simulink model "connected_tanks_simulink"  (R2020a)
settings: Solver=VariableStepAuto  StartTime=0.0  StopTime=300  RelTol=1e-3
values from neighbouring files (symbols this model uses):
  a1 = 1.78    [connected_tanks.m]
  A1 = 15.518    [connected_tanks.m]
  a2 = 1.78    [connected_tanks.m]
  A2 = 15.518    [connected_tanks.m]
  g = 981    [connected_tanks.m]
  K0 = 5    [connected_tanks.m]
  K1 = 5    [connected_tanks.m]
  Kd = 1    [connected_tanks.m]
  Ke = 1    [connected_tanks.m]
  Km = 4.6    [connected_tanks.m]
libraries: fuzblock x2, simulink x1
settings Model: Creator=paulo  LastModifiedBy=paulo

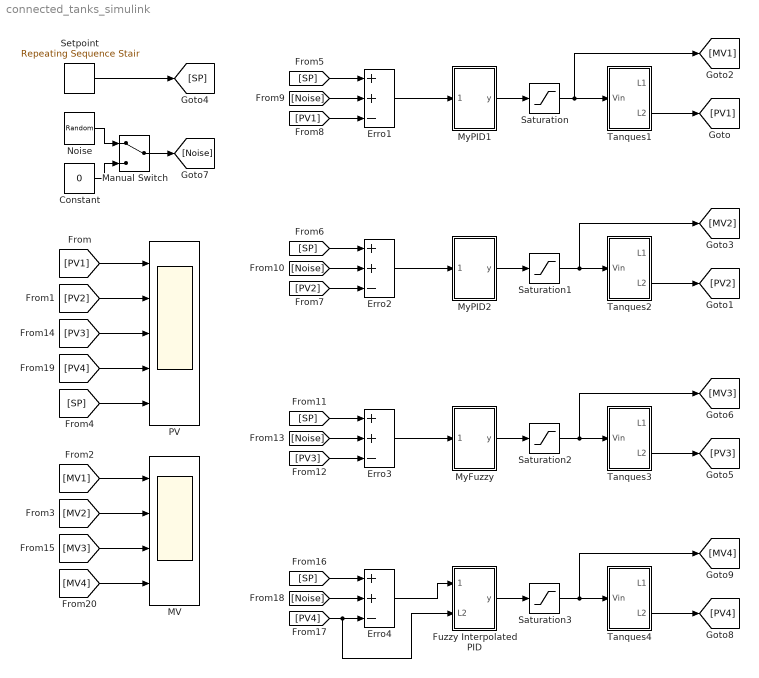
== system connected_tanks_simulink ==
  Constant : Constant  Value=0
  Erro{1..4} (4 alike) : Sum  Inputs=++-
  Fuzzy Interpolated PID : Subsystem
  MV : Scope  NumInputPorts=4
  Manual Switch : ManualSwitch
  MyFuzzy : Subsystem
  MyPID1 : Subsystem
  MyPID2 : Subsystem
  Noise : UniformRandomNumber  Minimum=-.5  Maximum=+.5  SampleTime=.5
  PV : Scope  NumInputPorts=5
  Saturation{,1..3} (4 alike) : Saturate  UpperLimit=120  LowerLimit=0
  Setpoint : simulink/Sources/Repeating Sequence Stair  OutValues=[5 20 15].'  tsamp=100  OutMin=[]  OutMax=[]  OutDataTypeStr=double  OutputDataTypeScalingMode=double  OutDataType=fixdt(0,8)  ConRadixGroup=Best Precision: Vector-wise  OutScaling=2^-12
  Tanques1 : Subsystem
  Tanques2 : Subsystem
  Tanques3 : Subsystem
  Tanques4 : Subsystem
  wires:
  Tanques1/2(L2) -> [PV1]
  Erro1/1 -> MyPID1/1(erro)
  MyPID1/1(y) -> Saturation/1
  Erro2/1 -> MyPID2/1(erro)
  Tanques2/2(L2) -> [PV2]
  [MV1] -> MV/1
  [MV2] -> MV/2
  Saturation/1 -> [MV1], Tanques1/1(Vin)
  Noise/1 -> Manual Switch/1
  Constant/1 -> Manual Switch/2
  MyPID2/1(y) -> Saturation1/1
  Saturation1/1 -> [MV2], Tanques2/1(Vin)
  Setpoint/1 -> [SP]
  [SP] -> Erro1/1
  [SP] -> Erro2/1
  Erro3/1 -> MyFuzzy/1(erro)
  MyFuzzy/1(y) -> Saturation2/1
  Tanques3/2(L2) -> [PV3]
  Saturation2/1 -> [MV3], Tanques3/1(Vin)
  [SP] -> Erro3/1
  [PV1] -> Erro1/3
  [Noise] -> Erro1/2
  Manual Switch/1 -> [Noise]
  [PV3] -> Erro3/3
  [Noise] -> Erro3/2
  [PV2] -> Erro2/3
  [Noise] -> Erro2/2
  [MV3] -> MV/3
  Tanques4/2(L2) -> [PV4]
  Saturation3/1 -> [MV4], Tanques4/1(Vin)
  [SP] -> Erro4/1
  Fuzzy Interpolated PID/1(y) -> Saturation3/1
  [PV4] -> Fuzzy Interpolated PID/2(L2), Erro4/3
  [Noise] -> Erro4/2
  Erro4/1 -> Fuzzy Interpolated PID/1(erro)
  [MV4] -> MV/4
  [PV1] -> PV/1
  [PV2] -> PV/2
  [PV3] -> PV/3
  [PV4] -> PV/4
  [SP] -> PV/5

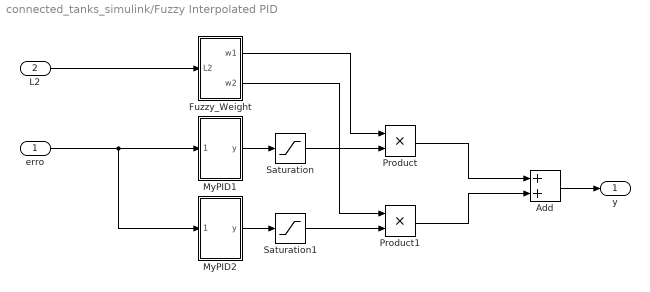
== system connected_tanks_simulink/Fuzzy Interpolated PID ==
  erro : Inport
  L2 : Inport  Port=2
  Add : Sum
  Fuzzy_Weight : Subsystem
  MyPID1 : Subsystem
  MyPID2 : Subsystem
  Product : Product
  Product1 : Product
  Saturation : Saturate  UpperLimit=120  LowerLimit=0
  Saturation1 : Saturate  UpperLimit=120  LowerLimit=0
  y : Outport
  wires:
  Add/1 -> y/1
  MyPID2/1(y) -> Saturation1/1
  MyPID1/1(y) -> Saturation/1
  erro/1 -> MyPID2/1(erro), MyPID1/1(erro)
  L2/1 -> Fuzzy_Weight/1(L2)
  Saturation/1 -> Product/2
  Saturation1/1 -> Product1/2
  Fuzzy_Weight/2(w2) -> Product1/1
  Fuzzy_Weight/1(w1) -> Product/1
  Product/1 -> Add/1
  Product1/1 -> Add/2

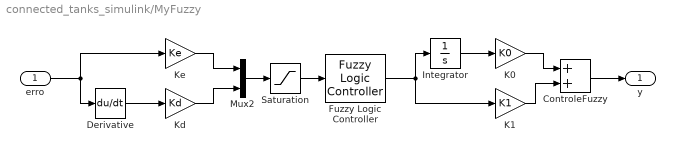
== system connected_tanks_simulink/MyFuzzy ==
  erro : Inport
  ControleFuzzy : Sum
  Derivative : Derivative
  Fuzzy Logic Controller : fuzblock/Fuzzy Logic  Controller  FIS=fuzzy_pid  OutputSampleNumber=101  DataType=double  FuzzifiedInputs=off  RuleFiringStrengths=off  RuleOutputs=off  AggregatedOutputs=off  SimulateUsing=Interpreted execution  OutOfRangeInputValueMessage=warning  NoRuleFiredMessage=warning  EmptyOutputFuzzySetMessage=warning
  Integrator : Integrator
  K0 : Gain  Gain=K0
  K1 : Gain  Gain=K1
  Kd : Gain  Gain=Kd
  Ke : Gain  Gain=Ke
  Mux2 : Mux  Inputs=2
  Saturation : Saturate  UpperLimit=1  LowerLimit=-1
  y : Outport
  wires:
  ControleFuzzy/1 -> y/1
  Integrator/1 -> K0/1
  Ke/1 -> Mux2/1
  Fuzzy Logic Controller/1 -> Integrator/1, K1/1
  Derivative/1 -> Kd/1
  Kd/1 -> Mux2/2
  K0/1 -> ControleFuzzy/1
  K1/1 -> ControleFuzzy/2
  Mux2/1 -> Saturation/1
  Saturation/1 -> Fuzzy Logic Controller/1
  erro/1 -> Ke/1, Derivative/1

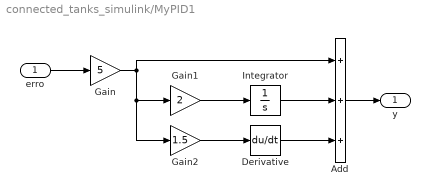
== system connected_tanks_simulink/MyPID1 ==
  erro : Inport
  Add : Sum  Inputs=+++
  Derivative : Derivative
  Gain : Gain  Gain=5
  Gain1 : Gain  Gain=2
  Gain2 : Gain  Gain=1.5
  Integrator : Integrator
  y : Outport
  wires:
  erro/1 -> Gain/1
  Gain/1 -> Gain2/1, Gain1/1, Add/1
  Gain1/1 -> Integrator/1
  Integrator/1 -> Add/2
  Gain2/1 -> Derivative/1
  Derivative/1 -> Add/3
  Add/1 -> y/1

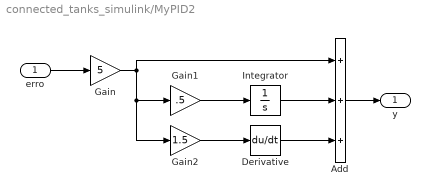
== system connected_tanks_simulink/MyPID2 ==
  erro : Inport
  Add : Sum  Inputs=+++
  Derivative : Derivative
  Gain : Gain  Gain=5
  Gain1 : Gain  Gain=.5
  Gain2 : Gain  Gain=1.5
  Integrator : Integrator
  y : Outport
  wires:
  erro/1 -> Gain/1
  Gain/1 -> Gain2/1, Gain1/1, Add/1
  Gain1/1 -> Integrator/1
  Integrator/1 -> Add/2
  Gain2/1 -> Derivative/1
  Derivative/1 -> Add/3
  Add/1 -> y/1

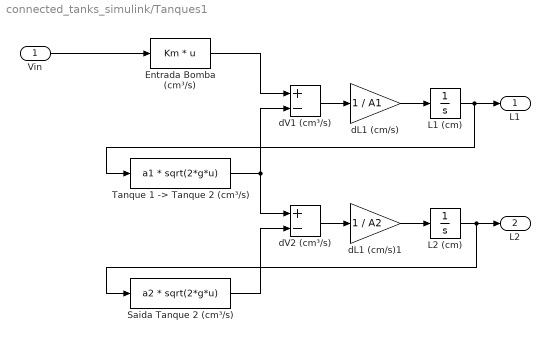
== system connected_tanks_simulink/Tanques1 ==
  Vin : Inport
  Entrada Bomba (cm³/s) : Fcn  Expr=Km * u
  L1 (cm) : Integrator
  L2 (cm) : Integrator
  Saida Tanque 2 (cm³/s) : Fcn  Expr=a2 * sqrt(2*g*u)
  "Tanque 1 -> Tanque 2 (cm³/s)" : Fcn  Expr=a1 * sqrt(2*g*u)
  dL1 (cm/s) : Gain  Gain=1 / A1
  dL1 (cm/s)1 : Gain  Gain=1 / A2
  dV1 (cm³/s) : Sum  Inputs=+-
  dV2 (cm³/s) : Sum  Inputs=+-
  L1 : Outport
  L2 : Outport  Port=2
  wires:
  Entrada Bomba (cm³/s)/1 -> dV1 (cm³/s)/1
  L2 (cm)/1 -> Saida Tanque 2 (cm³/s)/1, L2/1
  dV1 (cm³/s)/1 -> dL1 (cm/s)/1
  dV2 (cm³/s)/1 -> dL1 (cm/s)1/1
  Vin/1 -> Entrada Bomba (cm³/s)/1
  "Tanque 1 -> Tanque 2 (cm³/s)"/1 -> dV2 (cm³/s)/1, dV1 (cm³/s)/2
  L1 (cm)/1 -> L1/1, "Tanque 1 -> Tanque 2 (cm³/s)"/1
  Saida Tanque 2 (cm³/s)/1 -> dV2 (cm³/s)/2
  dL1 (cm/s)/1 -> L1 (cm)/1
  dL1 (cm/s)1/1 -> L2 (cm)/1

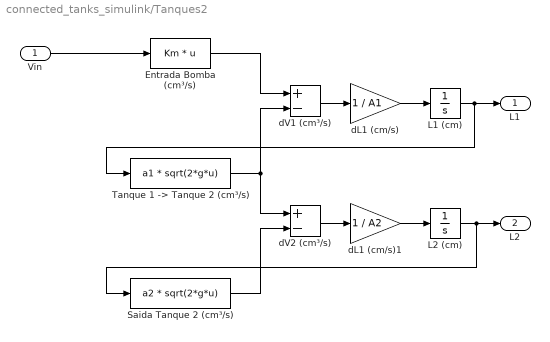
== system connected_tanks_simulink/Tanques2 ==
  Vin : Inport
  Entrada Bomba (cm³/s) : Fcn  Expr=Km * u
  L1 (cm) : Integrator
  L2 (cm) : Integrator
  Saida Tanque 2 (cm³/s) : Fcn  Expr=a2 * sqrt(2*g*u)
  "Tanque 1 -> Tanque 2 (cm³/s)" : Fcn  Expr=a1 * sqrt(2*g*u)
  dL1 (cm/s) : Gain  Gain=1 / A1
  dL1 (cm/s)1 : Gain  Gain=1 / A2
  dV1 (cm³/s) : Sum  Inputs=+-
  dV2 (cm³/s) : Sum  Inputs=+-
  L1 : Outport
  L2 : Outport  Port=2
  wires:
  Entrada Bomba (cm³/s)/1 -> dV1 (cm³/s)/1
  L2 (cm)/1 -> Saida Tanque 2 (cm³/s)/1, L2/1
  dV1 (cm³/s)/1 -> dL1 (cm/s)/1
  dV2 (cm³/s)/1 -> dL1 (cm/s)1/1
  Vin/1 -> Entrada Bomba (cm³/s)/1
  "Tanque 1 -> Tanque 2 (cm³/s)"/1 -> dV2 (cm³/s)/1, dV1 (cm³/s)/2
  L1 (cm)/1 -> L1/1, "Tanque 1 -> Tanque 2 (cm³/s)"/1
  Saida Tanque 2 (cm³/s)/1 -> dV2 (cm³/s)/2
  dL1 (cm/s)/1 -> L1 (cm)/1
  dL1 (cm/s)1/1 -> L2 (cm)/1

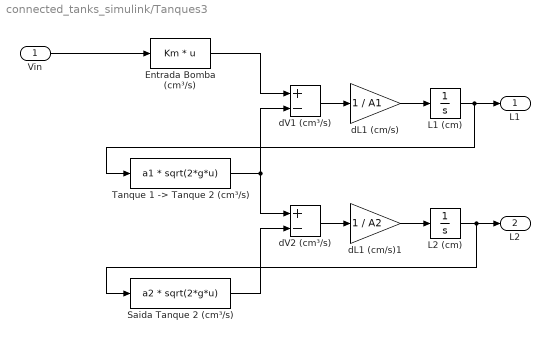
== system connected_tanks_simulink/Tanques3 ==
  Vin : Inport
  Entrada Bomba (cm³/s) : Fcn  Expr=Km * u
  L1 (cm) : Integrator
  L2 (cm) : Integrator
  Saida Tanque 2 (cm³/s) : Fcn  Expr=a2 * sqrt(2*g*u)
  "Tanque 1 -> Tanque 2 (cm³/s)" : Fcn  Expr=a1 * sqrt(2*g*u)
  dL1 (cm/s) : Gain  Gain=1 / A1
  dL1 (cm/s)1 : Gain  Gain=1 / A2
  dV1 (cm³/s) : Sum  Inputs=+-
  dV2 (cm³/s) : Sum  Inputs=+-
  L1 : Outport
  L2 : Outport  Port=2
  wires:
  Entrada Bomba (cm³/s)/1 -> dV1 (cm³/s)/1
  L2 (cm)/1 -> Saida Tanque 2 (cm³/s)/1, L2/1
  dV1 (cm³/s)/1 -> dL1 (cm/s)/1
  dV2 (cm³/s)/1 -> dL1 (cm/s)1/1
  Vin/1 -> Entrada Bomba (cm³/s)/1
  "Tanque 1 -> Tanque 2 (cm³/s)"/1 -> dV2 (cm³/s)/1, dV1 (cm³/s)/2
  L1 (cm)/1 -> L1/1, "Tanque 1 -> Tanque 2 (cm³/s)"/1
  Saida Tanque 2 (cm³/s)/1 -> dV2 (cm³/s)/2
  dL1 (cm/s)/1 -> L1 (cm)/1
  dL1 (cm/s)1/1 -> L2 (cm)/1

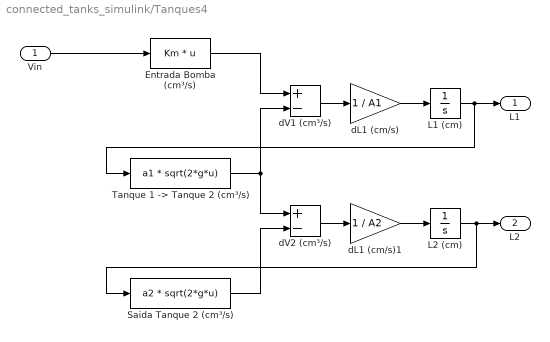
== system connected_tanks_simulink/Tanques4 ==
  Vin : Inport
  Entrada Bomba (cm³/s) : Fcn  Expr=Km * u
  L1 (cm) : Integrator
  L2 (cm) : Integrator
  Saida Tanque 2 (cm³/s) : Fcn  Expr=a2 * sqrt(2*g*u)
  "Tanque 1 -> Tanque 2 (cm³/s)" : Fcn  Expr=a1 * sqrt(2*g*u)
  dL1 (cm/s) : Gain  Gain=1 / A1
  dL1 (cm/s)1 : Gain  Gain=1 / A2
  dV1 (cm³/s) : Sum  Inputs=+-
  dV2 (cm³/s) : Sum  Inputs=+-
  L1 : Outport
  L2 : Outport  Port=2
  wires:
  Entrada Bomba (cm³/s)/1 -> dV1 (cm³/s)/1
  L2 (cm)/1 -> Saida Tanque 2 (cm³/s)/1, L2/1
  dV1 (cm³/s)/1 -> dL1 (cm/s)/1
  dV2 (cm³/s)/1 -> dL1 (cm/s)1/1
  Vin/1 -> Entrada Bomba (cm³/s)/1
  "Tanque 1 -> Tanque 2 (cm³/s)"/1 -> dV2 (cm³/s)/1, dV1 (cm³/s)/2
  L1 (cm)/1 -> L1/1, "Tanque 1 -> Tanque 2 (cm³/s)"/1
  Saida Tanque 2 (cm³/s)/1 -> dV2 (cm³/s)/2
  dL1 (cm/s)/1 -> L1 (cm)/1
  dL1 (cm/s)1/1 -> L2 (cm)/1

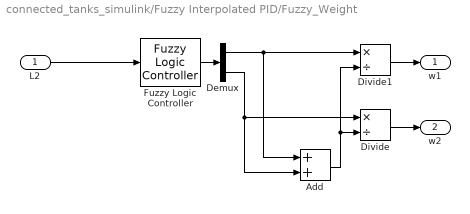
== system connected_tanks_simulink/Fuzzy Interpolated PID/Fuzzy_Weight ==
  L2 : Inport
  Add : Sum
  Demux : Demux  Outputs=2
  Divide : Product  Inputs=*/
  Divide1 : Product  Inputs=*/
  Fuzzy Logic Controller : fuzblock/Fuzzy Logic  Controller  FIS=fuzzy_ts_nivel  OutputSampleNumber=101  DataType=double  FuzzifiedInputs=off  RuleFiringStrengths=off  RuleOutputs=off  AggregatedOutputs=off  SimulateUsing=Interpreted execution  OutOfRangeInputValueMessage=warning  NoRuleFiredMessage=warning  EmptyOutputFuzzySetMessage=warning
  w1 : Outport
  w2 : Outport  Port=2
  wires:
  Demux/2 -> Divide/1, Add/2
  Fuzzy Logic Controller/1 -> Demux/1
  Add/1 -> Divide1/2, Divide/2
  L2/1 -> Fuzzy Logic Controller/1
  Demux/1 -> Add/1, Divide1/1
  Divide1/1 -> w1/1
  Divide/1 -> w2/1

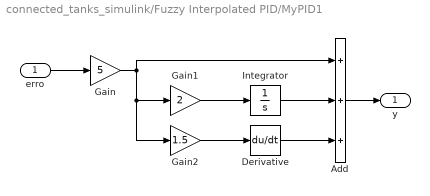
== system connected_tanks_simulink/Fuzzy Interpolated PID/MyPID1 ==
  erro : Inport
  Add : Sum  Inputs=+++
  Derivative : Derivative
  Gain : Gain  Gain=5
  Gain1 : Gain  Gain=2
  Gain2 : Gain  Gain=1.5
  Integrator : Integrator
  y : Outport
  wires:
  erro/1 -> Gain/1
  Gain/1 -> Gain2/1, Gain1/1, Add/1
  Gain1/1 -> Integrator/1
  Integrator/1 -> Add/2
  Gain2/1 -> Derivative/1
  Derivative/1 -> Add/3
  Add/1 -> y/1

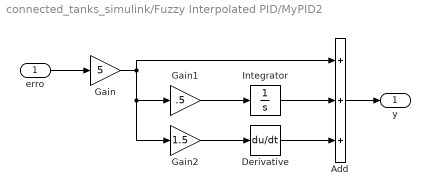
== system connected_tanks_simulink/Fuzzy Interpolated PID/MyPID2 ==
  erro : Inport
  Add : Sum  Inputs=+++
  Derivative : Derivative
  Gain : Gain  Gain=5
  Gain1 : Gain  Gain=.5
  Gain2 : Gain  Gain=1.5
  Integrator : Integrator
  y : Outport
  wires:
  erro/1 -> Gain/1
  Gain/1 -> Gain2/1, Gain1/1, Add/1
  Gain1/1 -> Integrator/1
  Integrator/1 -> Add/2
  Gain2/1 -> Derivative/1
  Derivative/1 -> Add/3
  Add/1 -> y/1
